simulink model "shipmoodel"  (R2017a)
settings: Solver=VariableStepAuto  StartTime=0.0  StopTime=1000.0  RelTol=1e-3
values from neighbouring files (symbols this model uses):
  b = 0.001    [Init.m]
  K = 0.1    [Init.m]
  K_d = 80    [Init.m]
  K_i = 0.5    [Init.m]
  K_p = 2    [Init.m]
  T = 20    [Init.m]
  U = 5    [Init.m]
settings Model: Creator=martimos  LastModifiedBy=martimos

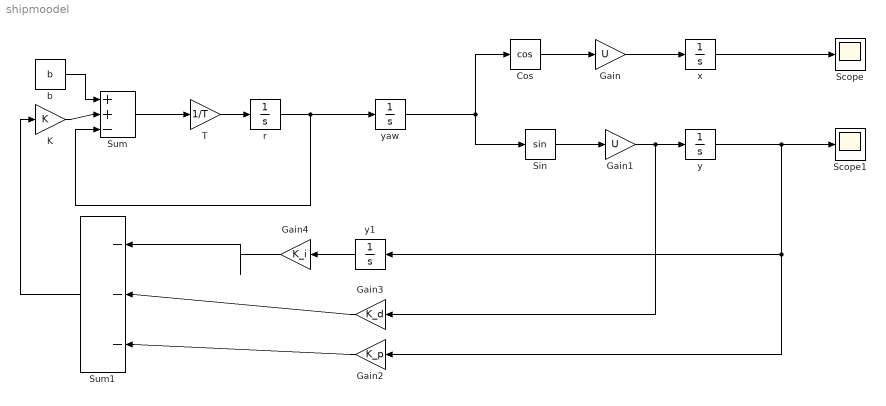
== system shipmoodel ==
  Cos : Trigonometry  Operator=cos
  Gain : Gain  Gain=U
  Gain1 : Gain  Gain=U
  Gain2 : Gain  Gain=K_p
  Gain3 : Gain  Gain=K_d
  Gain4 : Gain  Gain=K_i
  K : Gain  Gain=K
  Scope : Scope
  Scope1 : Scope
  Sin : Trigonometry
  Sum : Sum  Inputs=|++-
  Sum1 : Sum  Inputs=|---
  T : Gain  Gain=1/T
  b : Constant  Value=b
  r : Integrator
  x : Integrator
  y : Integrator
  y1 : Integrator
  yaw : Integrator
  wires:
  Gain/1 -> x/1
  Cos/1 -> Gain/1
  Gain1/1 -> Gain3/1, y/1
  Sin/1 -> Gain1/1
  yaw/1 -> Sin/1, Cos/1
  b/1 -> Sum/1
  K/1 -> Sum/2
  r/1 -> Sum/3, yaw/1
  Sum/1 -> T/1
  T/1 -> r/1
  Sum1/1 -> K/1
  y/1 -> Scope1/1, y1/1, Gain2/1
  Gain3/1 -> Sum1/2
  Gain2/1 -> Sum1/3
  y1/1 -> Gain4/1
  Gain4/1 -> Sum1/1
  x/1 -> Scope/1
